simulink model "Filter_attivo"  (R2016b)
settings: Solver=ode23t  StartTime=0.0  StopTime=2.4  MaxStep=1e-4  RelTol=1e-3  EnableMultiTasking=on
values from neighbouring files (symbols this model uses):
  ampiezza_rete = 150/sqrt(3)    [Data.m]    (also in taratura.m)
  C = 2.2e-3    (= 0.0022)    [Data.m]
  C_raddr = 600e-6    (= 0.0006)    [Data.m]
  f = 50    [Data.m]    (also in Spettro_complesso.m = bar(-fp((26:25:25000-25)),PyTHD(length(PyTHD)-1:-1:length(Py)
  f_am = 500    [Data.m]
  h = Lagrange_coef(f,1/Tc)    [Data.m]    (also in Lagrange_coef.m = NaN(4,round(fc/f1*0.5)))
  h_rit = Lagrange_coef_rit(1.5)    [Data.m]
  k_interno = 0.99    [tuning.m]
  k_par_AM = 10    [Data.m]
  ki_PI = 0.2    [Data.m]
  ki_PLL = 1000    [Data.m]
  ki_ris = 47.5*2    (= 95)    [Data.m]
  kp_PI = 1.57    [Data.m]
  kp_PLL = 0.9    [Data.m]
  kp_ris = 47.5*0.089*2    (= 8.455)    [Data.m]
  L_disaccoppiamento = 2*1.18e-3    (= 0.00236)    [Data.m]    (also in taratura.m)
  L_rete = 4e-3    (= 0.004)    [Data.m]    (also in tuning.m)
  max_PI = 8    [Data.m]
  max_PLL = 1000    [Data.m]
  min_PI = -8    [Data.m]
  min_PLL = -1000    [Data.m]
  Notch_z = 1-Peaking_z    [Data.m]
  Notch_z_AM1 = 1-Peaking_z_AM1    [Notch.m]
  peak_rete = Peaking(f,1/Tc,0.1)    [Data.m]
  Peaking_dir1_d = c2d(Peaking_dir1_s,1/fs,'tustin')    [semipeaking.m]
  pendenza = 1000    [Data.m]
  R_carico = 50    [Data.m]
  R_disaccoppiamento = 2*13e-3    (= 0.026)    [Data.m]    (also in taratura.m)
  R_raddr = 60    [Data.m]
  R_rete = 100e-3    (= 0.1)    [Data.m]    (also in tuning.m = 0.01)
  T = 20e-3    (= 0.02)    [Data.m]    (also in tuning.m)
  tau_filtro_Vdc_ref = 0.15    [Data.m]
  Tc = 1/10000    (= 0.0001)    [Data.m]    (also in taratura.m; tuning.m)
  Vdc_ref = 200    [Data.m]    (also in taratura.m)
  w_filtro = 2*pi*f_taglio    (= 56548.6677646)    [Data.m]
undefined symbols (not defined in the file or in its folder): DiscIntNeverNeededParam, k_par, k_ser, Notch_z_AM1_5, Notch_z_AM1_7, Notch_z_AM2_5, Notch_z_AM2_7, Peaking_inv_d, plecs, Q_inv
libraries: powerlib x54, simulink x8, powerlib_extras x4, powerlib_meascontrol x2
(part 3 of 5)

== system Filter_attivo/Controllo tensione/Controllo ripetitivo/Notch Prima Armonica/D ==
  ab(c) : Inport
  Gain : Gain  Gain=[1 0; 1/sqrt(3) 2/sqrt(3)]  Multiplication=Matrix(K*u)
  dq(0) : Outport
  wires:
  Gain/1 -> dq(0)/1
  ab(c)/1 -> Gain/1

== system Filter_attivo/Controllo tensione/Controllo ripetitivo/Notch Prima Armonica/Filtro notch prima armonica  ==
  ir : Inport
  Discrete Transfer Fcn : DiscreteTransferFcn  Numerator=Notch_z.num{1,1}  Denominator=Notch_z.den{1,1}
  irh : Outport
  wires:
  ir/1 -> Discrete Transfer Fcn/1
  Discrete Transfer Fcn/1 -> irh/1

== system Filter_attivo/Controllo tensione/Controllo ripetitivo/Notch Prima Armonica/Filtro notch prima armonica 1 ==
  ir : Inport
  Discrete Transfer Fcn : DiscreteTransferFcn  Numerator=Notch_z.num{1,1}  Denominator=Notch_z.den{1,1}
  irh : Outport
  wires:
  Discrete Transfer Fcn/1 -> irh/1
  ir/1 -> Discrete Transfer Fcn/1

== system Filter_attivo/Rete/generatore diretta e inversa/Scope1/ InputMux  ==
  In1 : Inport
  Convert1 : DataTypeConversion  SaturateOnIntegerOverflow=on  RndMeth=Zero
  Mux : Mux  Inputs=1
  Out : Outport
  wires:
  Mux/1 -> Out/1
  In1/1 -> Convert1/1
  Convert1/1 -> Mux/1

== system Filter_attivo/Controllo tensione/Controllo PR 10 kHz/Controllo risonante/Contributo controllo risonante fondamentale/PIR_tustin_prewarp ==
  errore_d : Inport
  errore_q : Inport  Port=2
  Vdc : Inport  Port=3
  Enable : EnablePort  StatesWhenEnabling=reset
  Constant : Constant  Value=kp_ris
  Constant1 : Constant  Value=kr_ris
  Constant2 : Constant  Value=Tc
  Constant3 : Constant  Value=delta
  Constant4 : Constant  Value=w_ris
  Gain : Gain  Gain=-1
  MATLAB Function : MATLAB Function  TreatAsAtomicUnit=on
  MATLAB Function1 : MATLAB Function  TreatAsAtomicUnit=on
  vf1_d : Outport
  vfq_q : Outport  Port=2
  wires:
  errore_d/1 -> MATLAB Function/1(error)
  Constant/1 -> MATLAB Function1/2(kp), MATLAB Function/2(kp)
  Constant1/1 -> MATLAB Function1/3(ki), MATLAB Function/3(ki)
  Vdc/1 -> Gain/1, MATLAB Function1/5(max), MATLAB Function/5(max)
  Gain/1 -> MATLAB Function1/4(min), MATLAB Function/4(min)
  Constant2/1 -> MATLAB Function1/6(Tc), MATLAB Function/6(Tc)
  Constant3/1 -> MATLAB Function1/7(delta), MATLAB Function/7(delta)
  Constant4/1 -> MATLAB Function/8(w0)
  MATLAB Function/1(out) -> vf1_d/1
  MATLAB Function1/1(out) -> vfq_q/1
  errore_q/1 -> MATLAB Function1/8(w0), MATLAB Function1/1(error)

== system Filter_attivo/Controllo tensione/Controllo PR 10 kHz/Controllo risonante/Contributo controllo risonante fondamentale/PI_risonante ==
  note: Questa è la discretizzazione di un PIR alla frequenza w0 della fondamentale (314 rad/s)
      | utlizzando la discretizzazione di Tustin con Prewarp
  In1 : Inport
  In2 : Inport  Port=2
  Enable : EnablePort  StatesWhenEnabling=reset
  Add : Sum
  Demux : Demux  Outputs=2
  Demux1 : Demux  Outputs=2
  Discrete Transfer Fcn2 : DiscreteTransferFcn  Numerator=[sin(Tc*2*pi*f) 0 -sin(Tc*2*pi*f)]  Denominator=[2*2*pi*f -2*2*2*pi*f*cos(Tc*2*pi*f) 2*2*pi*f]
  Discrete Transfer Fcn3 : DiscreteTransferFcn  Numerator=[sin(Tc*2*pi*f) 0 -sin(Tc*2*pi*f)]  Denominator=[2*2*pi*f -2*2*2*pi*f*cos(Tc*2*pi*f) 2*2*pi*f]
  Gain : Gain  Gain=ki_ris
  Gain1 : Gain  Gain=kp_ris
  Mux : Mux  Inputs=2
  Mux1 : Mux  Inputs=2
  Out1 : Outport
  Out2 : Outport  Port=2
  wires:
  Mux/1 -> Gain1/1, Gain/1
  In1/1 -> Mux/1
  In2/1 -> Mux/2
  Demux/1 -> Out1/1
  Demux/2 -> Out2/1
  Add/1 -> Demux/1
  Mux1/1 -> Add/2
  Gain/1 -> Demux1/1
  Gain1/1 -> Add/1
  Demux1/1 -> Discrete Transfer Fcn2/1
  Demux1/2 -> Discrete Transfer Fcn3/1
  Discrete Transfer Fcn2/1 -> Mux1/1
  Discrete Transfer Fcn3/1 -> Mux1/2

== system Filter_attivo/Controllo tensione/Controllo PR 10 kHz/Controllo risonante/FILTRO peaking inversa_prima/Scope ==
  1 : Inport
  " InputMux " : Subsystem
      mask Display: disp('Mux')
  " S-Function " : S-Function  FunctionName=plecs  SFunctionDeploymentMode=off  EnableBusSupport=off
  wires:
  1/1 -> " InputMux "/1(In1)
  " InputMux "/1(Out) -> " S-Function "/1

== system Filter_attivo/Controllo tensione/Controllo PR 10 kHz/PLL_tempo_discreto/Subsystem/FILTRO peaking diretta_prima ==
  In2 : Inport
  Demux : Demux  Outputs=2
  Discrete Transfer Fcn : DiscreteTransferFcn  Numerator=cell2mat(Peaking_dir1_d(1,1).Num)  Denominator=cell2mat(Peaking_dir1_d(1,1).Den)
  Discrete Transfer Fcn1 : DiscreteTransferFcn  Numerator=cell2mat(Peaking_dir1_d(1,2).Num)  Denominator=cell2mat(Peaking_dir1_d(1,2).Den)
  Discrete Transfer Fcn2 : DiscreteTransferFcn  Numerator=cell2mat(Peaking_dir1_d(2,1).Num)  Denominator=cell2mat(Peaking_dir1_d(2,1).Den)
  Discrete Transfer Fcn3 : DiscreteTransferFcn  Numerator=cell2mat(Peaking_dir1_d(2,2).Num)  Denominator=cell2mat(Peaking_dir1_d(2,2).Den)
  Mux1 : Mux  Inputs=2
  Scope : Subsystem  LoadFcn=plecs('sl', 300);  InitFcn=plecs('sl', 314);  StartFcn=plecs('sl', 308);  StopFcn=plecs('sl', 309);  mask{Settings=<binary blob, 216 chars, not shown>}
      mask init:
      | plecs('sl', 315);
      settings: CopyFcn=plecs('sl', 303);  DeleteFcn=plecs('sl', 305);  UndoDeleteFcn=plecs('sl', 306);  PreSaveFcn=plecs('sl', 311);  NameChangeFcn=plecs('sl', 310);  DestroyFcn=plecs('sl', 307);  OpenFcn=plecs('sl', 302);  ErrorFcn=plerrorfcn
      mask Display: plot([0.1 0.9 0.9 0.1 0.1], [0.9 0.9 0.5 0.5 0.9])
  Sum3 : Sum  Inputs=|++
  Sum4 : Sum  Inputs=|++
  Out1 : Outport
  wires:
  Demux/1 -> Discrete Transfer Fcn2/1, Discrete Transfer Fcn/1
  Demux/2 -> Discrete Transfer Fcn1/1, Discrete Transfer Fcn3/1
  Discrete Transfer Fcn2/1 -> Sum4/1
  Sum4/1 -> Mux1/2
  Mux1/1 -> Out1/1
  Sum3/1 -> Mux1/1, Scope/1(1)
  Discrete Transfer Fcn/1 -> Sum3/1
  Discrete Transfer Fcn1/1 -> Sum3/2
  In2/1 -> Demux/1
  Discrete Transfer Fcn3/1 -> Sum4/2

== system Filter_attivo/Controllo tensione/Controllo PR 10 kHz/PLL_tempo_discreto/Subsystem/notch_prima_tensione ==
  In1 : Inport
  FILTRO peaking diretta_prima : Subsystem
  Sum : Sum  Inputs=|+-
  Out1 : Outport
  wires:
  In1/1 -> FILTRO peaking diretta_prima/1(In2), Sum/1
  Sum/1 -> Out1/1
  FILTRO peaking diretta_prima/1(Out1) -> Sum/2

== system Filter_attivo/Controllo tensione/Controllo PR 10 kHz/controllo /Scope/ InputMux  ==
  In1 : Inport
  Convert1 : DataTypeConversion  SaturateOnIntegerOverflow=on  RndMeth=Zero
  Mux : Mux  Inputs=1
  Out : Outport
  wires:
  Convert1/1 -> Mux/1
  In1/1 -> Convert1/1
  Mux/1 -> Out/1

== system Filter_attivo/Controllo tensione/Controllo PR 10 kHz/controllo /Scope1/ InputMux  ==
  In1 : Inport
  Convert1 : DataTypeConversion  SaturateOnIntegerOverflow=on  RndMeth=Zero
  Mux : Mux  Inputs=1
  Out : Outport
  wires:
  Mux/1 -> Out/1
  In1/1 -> Convert1/1
  Convert1/1 -> Mux/1

== system Filter_attivo/Controllo tensione/Controllo PR 10 kHz/controllo /Scope2/ InputMux  ==
  In1 : Inport
  Convert1 : DataTypeConversion  SaturateOnIntegerOverflow=on  RndMeth=Zero
  Mux : Mux  Inputs=1
  Out : Outport
  wires:
  Convert1/1 -> Mux/1
  In1/1 -> Convert1/1
  Mux/1 -> Out/1

== system Filter_attivo/Controllo tensione/Controllo PR 10 kHz/controllo /Scope3/ InputMux  ==
  In1 : Inport
  Convert1 : DataTypeConversion  SaturateOnIntegerOverflow=on  RndMeth=Zero
  Mux : Mux  Inputs=1
  Out : Outport
  wires:
  Mux/1 -> Out/1
  In1/1 -> Convert1/1
  Convert1/1 -> Mux/1

== system Filter_attivo/Controllo tensione/Controllo ripetitivo/Controllo ripetitivo/Regolatore ripetitivo/ Ripetitivo sincrono ==
  note: A
  ir : Inport
  Add : Sum
  Delay1 : Delay  DelayLength=rit
  Delay2 : Delay  DelayLength=round((1/ro/f/Tc)-rit-1)
  Gain1 : Gain
  Gain2 : Gain  Gain=k_ser_
  Scope : Subsystem  LoadFcn=plecs('sl', 300);  InitFcn=plecs('sl', 314);  StartFcn=plecs('sl', 308);  StopFcn=plecs('sl', 309);  mask{Settings=<binary blob, 384 chars, not shown>}
      mask init:
      | plecs('sl', 315);
      settings: CopyFcn=plecs('sl', 303);  DeleteFcn=plecs('sl', 305);  UndoDeleteFcn=plecs('sl', 306);  PreSaveFcn=plecs('sl', 311);  NameChangeFcn=plecs('sl', 310);  DestroyFcn=plecs('sl', 307);  OpenFcn=plecs('sl', 302);  ErrorFcn=plerrorfcn
      mask Display: plot([0.1 0.9 0.9 0.1 0.1], [0.9 0.9 0.5 0.5 0.9])
  Sum : Sum  Inputs=|--
  ritardo di 1.5 : DiscreteFir  Coefficients=[0.5 0. 0.5]
  Out : Outport
  wires:
  Gain2/1 -> Scope/2(2), Add/2
  Add/1 -> Scope/3(3), Out/1
  Delay1/1 -> Gain1/1
  Delay2/1 -> ritardo di 1.5/1
  Sum/1 -> Delay2/1
  Gain1/1 -> Sum/2
  ritardo di 1.5/1 -> Gain2/1, Delay1/1
  ir/1 -> Add/1, Sum/1

== system Filter_attivo/Controllo tensione/Controllo ripetitivo/Controllo ripetitivo/Regolatore ripetitivo/ Ripetitivo sincrono feedforward ==
  note: B
  note: A
  ir : Inport
  Delay2 : Delay  DelayLength=round((1/ro/f/Tc)-1)
  Delay3 : Delay  DelayLength=round((1/f/Tc/ro)-rit)
  Gain2 : Gain  Gain=k_ser_
  Q : DiscreteFir  Coefficients=[0.25 0.5 0.25]
  Sum : Sum  Inputs=|--
  Sum1 : Sum  Inputs=+-|
  Sum2 : Sum
  Out : Outport
  wires:
  Sum2/1 -> Out/1
  Gain2/1 -> Sum2/2
  Delay3/1 -> Gain2/1
  Sum1/1 -> Delay3/1
  ir/1 -> Sum/1, Sum2/1
  Q/1 -> Sum1/2, Sum/2
  Delay2/1 -> Q/1
  Sum/1 -> Delay2/1, Sum1/1

== system Filter_attivo/Controllo tensione/Controllo ripetitivo/Controllo ripetitivo/Regolatore ripetitivo/ buffer intero fase zero ==
  note: A
  e : Inport
  Add : Sum
  Delay1 : Delay  DelayLength=rit
  Delay2 : Delay  DelayLength=round((1/ro/f/Tc)-1-rit)
  Gain1 : Gain
  Gain2 : Gain  Gain=k_serie
  Q : DiscreteFir  Coefficients=[0.05 0.9 0.05]
  Scope : Subsystem  LoadFcn=plecs('sl', 300);  InitFcn=plecs('sl', 314);  StartFcn=plecs('sl', 308);  StopFcn=plecs('sl', 309);  mask{Settings=<binary blob, 424 chars, not shown>}
      mask init:
      | plecs('sl', 315);
      settings: CopyFcn=plecs('sl', 303);  DeleteFcn=plecs('sl', 305);  UndoDeleteFcn=plecs('sl', 306);  PreSaveFcn=plecs('sl', 311);  NameChangeFcn=plecs('sl', 310);  DestroyFcn=plecs('sl', 307);  OpenFcn=plecs('sl', 302);  ErrorFcn=plerrorfcn
      mask Display: plot([0.1 0.9 0.9 0.1 0.1], [0.9 0.9 0.5 0.5 0.9])
  Subsystem : Subsystem  mask{f_disturbo=265, g_disturbo=0.1}
      mask prompts: f_disturbo "frequeza [Hz] del disturbo"; g_disturbo "valore [pu] del disturbo"
  Sum : Sum  Inputs=|++
  Out : Outport
  wires:
  Gain1/1 -> Sum/2
  Sum/1 -> Delay2/1
  Delay2/1 -> Q/1
  Delay1/1 -> Gain1/1
  e/1 -> Subsystem/1(errore)
  Add/1 -> Out/1, Scope/3(3)
  Gain2/1 -> Scope/2(2), Add/2
  Subsystem/1(errore+disturbo) -> Scope/1(1), Sum/1, Add/1
  Q/1 -> Delay1/1, Gain2/1

== system Filter_attivo/Controllo tensione/Controllo ripetitivo/Controllo ripetitivo/Regolatore ripetitivo/ buffer intero fase zero1 ==
  note: A
  e : Inport
  Add : Sum
  Delay2 : Delay  DelayLength=round((1/ro/f/Tc)-4)
  Gain1 : Gain
  Gain2 : Gain  Gain=k_serie
  Q : DiscreteFir  Coefficients=[0.05 0.9 0.05]
  Q1 : DiscreteFir  Coefficients=[-0.0625 0.5625 0.5625 -0.0625]
  Q2 : DiscreteFir  Coefficients=[-0.0625 0.5625 0.5625 -0.0625]
  Scope : Subsystem  LoadFcn=plecs('sl', 300);  InitFcn=plecs('sl', 314);  StartFcn=plecs('sl', 308);  StopFcn=plecs('sl', 309);  mask{Settings=<binary blob, 424 chars, not shown>}
      mask init:
      | plecs('sl', 315);
      settings: CopyFcn=plecs('sl', 303);  DeleteFcn=plecs('sl', 305);  UndoDeleteFcn=plecs('sl', 306);  PreSaveFcn=plecs('sl', 311);  NameChangeFcn=plecs('sl', 310);  DestroyFcn=plecs('sl', 307);  OpenFcn=plecs('sl', 302);  ErrorFcn=plerrorfcn
      mask Display: plot([0.1 0.9 0.9 0.1 0.1], [0.9 0.9 0.5 0.5 0.9])
  Sum : Sum  Inputs=|++
  Out : Outport
  wires:
  Q/1 -> Q2/1
  e/1 -> Sum/1, Scope/1(1), Add/1
  Gain2/1 -> Add/2, Scope/2(2)
  Add/1 -> Scope/3(3), Out/1
  Q1/1 -> Gain1/1
  Delay2/1 -> Q/1
  Sum/1 -> Delay2/1
  Gain1/1 -> Sum/2
  Q2/1 -> Q1/1, Gain2/1

== system Filter_attivo/Controllo tensione/Controllo ripetitivo/Controllo ripetitivo/Regolatore ripetitivo/ buffer intero feedforward ==
  note: A
  note: B
  e : Inport
  Delay 1 : Delay  DelayLength=round((1/ro/f/Tc)-1)
  Delay 2 : Delay  DelayLength=round((1/ro/f/Tc)-rit)
  Gain2 : Gain  Gain=k_serie
  Q : DiscreteFir  Coefficients=[0.05 0.9 0.05]
  Scope : Subsystem  LoadFcn=plecs('sl', 300);  InitFcn=plecs('sl', 314);  StartFcn=plecs('sl', 308);  StopFcn=plecs('sl', 309);  mask{Settings=<binary blob, 892 chars, not shown>}
      mask init:
      | plecs('sl', 315);
      settings: CopyFcn=plecs('sl', 303);  DeleteFcn=plecs('sl', 305);  UndoDeleteFcn=plecs('sl', 306);  PreSaveFcn=plecs('sl', 311);  NameChangeFcn=plecs('sl', 310);  DestroyFcn=plecs('sl', 307);  OpenFcn=plecs('sl', 302);  ErrorFcn=plerrorfcn
      mask Display: plot([0.1 0.9 0.9 0.1 0.1], [0.9 0.9 0.5 0.5 0.9])
  Scope1 : Subsystem  LoadFcn=plecs('sl', 300);  InitFcn=plecs('sl', 314);  StartFcn=plecs('sl', 308);  StopFcn=plecs('sl', 309);  mask{Settings=<binary blob, 892 chars, not shown>}
      mask init:
      | plecs('sl', 315);
      settings: CopyFcn=plecs('sl', 303);  DeleteFcn=plecs('sl', 305);  UndoDeleteFcn=plecs('sl', 306);  PreSaveFcn=plecs('sl', 311);  NameChangeFcn=plecs('sl', 310);  DestroyFcn=plecs('sl', 307);  OpenFcn=plecs('sl', 302);  ErrorFcn=plerrorfcn
      mask Display: plot([0.1 0.9 0.9 0.1 0.1], [0.9 0.9 0.5 0.5 0.9])
  Subsystem : Subsystem  mask{f_disturbo=275, g_disturbo=0.3}
      mask prompts: f_disturbo "frequeza [Hz] del disturbo"; g_disturbo "valore [pu] del disturbo"
  Sum : Sum  Inputs=|++
  Sum1 : Sum  Inputs=++|
  Sum2 : Sum
  Out : Outport
  wires:
  Sum/1 -> Sum1/1, Delay 1/1
  Delay 1/1 -> Q/1
  Q/1 -> Sum/2, Sum1/2
  e/1 -> Scope1/1(1), Subsystem/1(errore)
  Sum1/1 -> Delay 2/1
  Delay 2/1 -> Gain2/1
  Gain2/1 -> Sum2/2
  Sum2/1 -> Out/1
  Subsystem/1(errore+disturbo) -> Sum2/1, Sum/1, Scope/1(1)

== system Filter_attivo/Controllo tensione/Controllo ripetitivo/Controllo ripetitivo/Regolatore ripetitivo/ buffer metà fase zero ==
  note: A
  e : Inport
  Add : Sum
  Delay1 : Delay  DelayLength=rit
  Delay2 : Delay  DelayLength=round((1/ro/f/Tc)-1-rit)
  Gain1 : Gain
  Gain2 : Gain  Gain=k_serie
  Q : DiscreteFir  Coefficients=[0.05 0.9 0.05]
  Scope : Subsystem  LoadFcn=plecs('sl', 300);  InitFcn=plecs('sl', 314);  StartFcn=plecs('sl', 308);  StopFcn=plecs('sl', 309);  mask{Settings=<binary blob, 424 chars, not shown>}
      mask init:
      | plecs('sl', 315);
      settings: CopyFcn=plecs('sl', 303);  DeleteFcn=plecs('sl', 305);  UndoDeleteFcn=plecs('sl', 306);  PreSaveFcn=plecs('sl', 311);  NameChangeFcn=plecs('sl', 310);  DestroyFcn=plecs('sl', 307);  OpenFcn=plecs('sl', 302);  ErrorFcn=plerrorfcn
      mask Display: plot([0.1 0.9 0.9 0.1 0.1], [0.9 0.9 0.5 0.5 0.9])
  Sum : Sum  Inputs=|--
  Out : Outport
  wires:
  Gain1/1 -> Sum/2
  Sum/1 -> Delay2/1
  Delay2/1 -> Q/1
  Delay1/1 -> Gain1/1
  e/1 -> Scope/1(1), Sum/1, Add/1
  Add/1 -> Out/1, Scope/3(3)
  Q/1 -> Gain2/1, Delay1/1
  Gain2/1 -> Scope/2(2), Add/2

== system Filter_attivo/Controllo tensione/Controllo ripetitivo/Controllo ripetitivo/Regolatore ripetitivo/ buffer metà feedforward ==
  note: A
  note: B
  e : Inport
  Delay2 : Delay  DelayLength=round((1/ro/f/Tc)-1)
  Delay3 : Delay  DelayLength=round((1/f/Tc/ro)-rit)
  Gain2 : Gain  Gain=k_serie
  Q : DiscreteFir  Coefficients=[0.05 0.9 0.05]
  Scope : Subsystem  LoadFcn=plecs('sl', 300);  InitFcn=plecs('sl', 314);  StartFcn=plecs('sl', 308);  StopFcn=plecs('sl', 309);  mask{Settings=<binary blob, 876 chars, not shown>}
      mask init:
      | plecs('sl', 315);
      settings: CopyFcn=plecs('sl', 303);  DeleteFcn=plecs('sl', 305);  UndoDeleteFcn=plecs('sl', 306);  PreSaveFcn=plecs('sl', 311);  NameChangeFcn=plecs('sl', 310);  DestroyFcn=plecs('sl', 307);  OpenFcn=plecs('sl', 302);  ErrorFcn=plerrorfcn
      mask Display: plot([0.1 0.9 0.9 0.1 0.1], [0.9 0.9 0.5 0.5 0.9])
  Subsystem : Subsystem  mask{f_disturbo=275, g_disturbo=0.1}
      mask prompts: f_disturbo "frequeza [Hz] del disturbo"; g_disturbo "valore [pu] del disturbo"
  Sum : Sum  Inputs=|--
  Sum1 : Sum  Inputs=+-|
  Sum2 : Sum
  Out : Outport
  wires:
  Sum2/1 -> Out/1
  Gain2/1 -> Sum2/2
  Delay3/1 -> Gain2/1
  Sum1/1 -> Delay3/1
  Q/1 -> Sum/2, Sum1/2
  Delay2/1 -> Q/1
  Sum/1 -> Delay2/1, Sum1/1
  Subsystem/1(errore+disturbo) -> Sum2/1, Sum/1, Scope/1(1)
  e/1 -> Subsystem/1(errore)

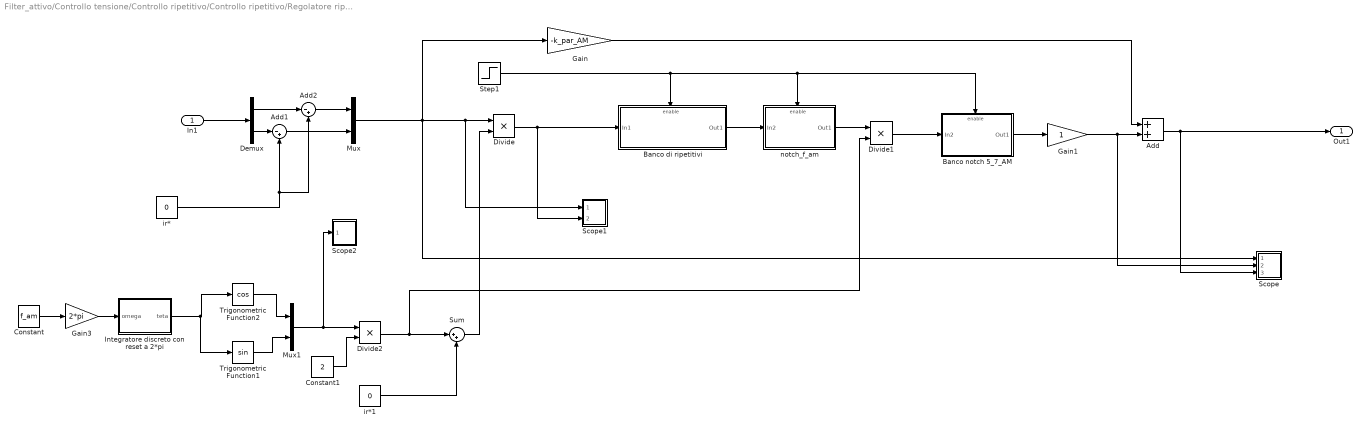
== system Filter_attivo/Controllo tensione/Controllo ripetitivo/Controllo ripetitivo/Regolatore ripetitivo/Ripetitivo Modulazione AM ==
  In1 : Inport
  Add : Sum
  Add1 : Sum  Inputs=|-+
  Add2 : Sum  Inputs=|-+
  Banco di ripetitivi : Subsystem
  Banco notch 5_7_AM : Subsystem
  Constant : Constant  Value=f_am
  Constant1 : Constant  Value=2
  Demux : Demux  Outputs=2
  Divide : Product  Inputs=**
  Divide1 : Product  Inputs=**
  Divide2 : Product  Inputs=**
  Gain : Gain  Gain=-k_par_AM
  Gain1 : Gain
  Gain3 : Gain  Gain=2*pi
  Integratore discreto con reset a 2*pi : Subsystem
  Mux : Mux  Inputs=2
  Mux1 : Mux  Inputs=2
  Scope : Subsystem  LoadFcn=plecs('sl', 300);  InitFcn=plecs('sl', 314);  StartFcn=plecs('sl', 308);  StopFcn=plecs('sl', 309);  mask{Settings=<binary blob, 424 chars, not shown>}
      mask init:
      | plecs('sl', 315);
      settings: CopyFcn=plecs('sl', 303);  DeleteFcn=plecs('sl', 305);  UndoDeleteFcn=plecs('sl', 306);  PreSaveFcn=plecs('sl', 311);  NameChangeFcn=plecs('sl', 310);  DestroyFcn=plecs('sl', 307);  OpenFcn=plecs('sl', 302);  ErrorFcn=plerrorfcn
      mask Display: plot([0.1 0.9 0.9 0.1 0.1], [0.9 0.9 0.5 0.5 0.9])
  Scope1 : Subsystem  LoadFcn=plecs('sl', 300);  InitFcn=plecs('sl', 314);  StartFcn=plecs('sl', 308);  StopFcn=plecs('sl', 309);  mask{Settings=<binary blob, 300 chars, not shown>}
      mask init:
      | plecs('sl', 315);
      settings: CopyFcn=plecs('sl', 303);  DeleteFcn=plecs('sl', 305);  UndoDeleteFcn=plecs('sl', 306);  PreSaveFcn=plecs('sl', 311);  NameChangeFcn=plecs('sl', 310);  DestroyFcn=plecs('sl', 307);  OpenFcn=plecs('sl', 302);  ErrorFcn=plerrorfcn
      mask Display: plot([0.1 0.9 0.9 0.1 0.1], [0.9 0.9 0.5 0.5 0.9])
  Scope2 : Subsystem  LoadFcn=plecs('sl', 300);  InitFcn=plecs('sl', 314);  StartFcn=plecs('sl', 308);  StopFcn=plecs('sl', 309);  mask{Settings=<binary blob, 216 chars, not shown>}
      mask init:
      | plecs('sl', 315);
      settings: CopyFcn=plecs('sl', 303);  DeleteFcn=plecs('sl', 305);  UndoDeleteFcn=plecs('sl', 306);  PreSaveFcn=plecs('sl', 311);  NameChangeFcn=plecs('sl', 310);  DestroyFcn=plecs('sl', 307);  OpenFcn=plecs('sl', 302);  ErrorFcn=plerrorfcn
      mask Display: plot([0.1 0.9 0.9 0.1 0.1], [0.9 0.9 0.5 0.5 0.9])
  Step1 : Step  Time=0.45
  Sum : Sum  Inputs=|++
  Trigonometric Function1 : Trigonometry
  Trigonometric Function2 : Trigonometry  Operator=cos
  ir* : Constant  Value=0
  ir*1 : Constant  Value=0
  notch_f_am : Subsystem
  Out1 : Outport
  wires:
  Gain/1 -> Add/1
  Constant/1 -> Gain3/1
  Gain3/1 -> Integratore discreto con reset a 2*pi/1(omega)
  Add1/1 -> Mux/2
  ir*/1 -> Add1/2, Add2/2
  Add/1 -> Out1/1, Scope/3(3)
  Demux/1 -> Add2/1
  In1/1 -> Demux/1
  Add2/1 -> Mux/1
  Demux/2 -> Add1/1
  Mux/1 -> Scope/1(1), Gain/1, Scope1/1(1), Divide/1
  Divide1/1 -> Banco notch 5_7_AM/1(In2)
  Banco notch 5_7_AM/1(Out1) -> Gain1/1
  Integratore discreto con reset a 2*pi/1(teta) -> Trigonometric Function1/1, Trigonometric Function2/1
  Trigonometric Function2/1 -> Mux1/1
  Trigonometric Function1/1 -> Mux1/2
  Mux1/1 -> Scope2/1(1), Divide2/1
  Constant1/1 -> Divide2/2
  Step1/1 -> notch_f_am/Enable, Banco notch 5_7_AM/Enable, Banco di ripetitivi/Enable
  Gain1/1 -> Scope/2(2), Add/2
  Divide/1 -> Banco di ripetitivi/1(In1), Scope1/2(2)
  Divide2/1 -> Divide1/2, Sum/1
  ir*1/1 -> Sum/2
  Sum/1 -> Divide/2
  Banco di ripetitivi/1(Out1) -> notch_f_am/1(In2)
  notch_f_am/1(Out1) -> Divide1/1

== system Filter_attivo/Controllo tensione/Controllo ripetitivo/Controllo ripetitivo/Regolatore ripetitivo/Scope ==
  1 : Inport
  " InputMux " : Subsystem
      mask Display: disp('Mux')
  " S-Function " : S-Function  FunctionName=plecs  SFunctionDeploymentMode=off  EnableBusSupport=off
  wires:
  1/1 -> " InputMux "/1(In1)
  " InputMux "/1(Out) -> " S-Function "/1

== system Filter_attivo/Controllo tensione/Controllo ripetitivo/Controllo ripetitivo/Regolatore ripetitivo/T ==
  dq : Inport
  teta : Inport  Port=2
  Demux : Demux  Outputs=2
  Fcn : Fcn  Expr=cos(u[3])*u[1]+sin(u[3])*u[2]
  Fcn1 : Fcn  Expr=-sin(u[3])*u[1]+cos(u[3])*u[2]
  Gain8 : Gain
  Mux : Mux  Inputs=3
  Mux1 : Mux  Inputs=2
  dq(teta) : Outport
  wires:
  dq/1 -> Demux/1
  Demux/1 -> Mux/1
  Demux/2 -> Mux/2
  Mux/1 -> Fcn/1, Fcn1/1
  Fcn/1 -> Mux1/1
  Fcn1/1 -> Mux1/2
  Mux1/1 -> dq(teta)/1
  teta/1 -> Gain8/1
  Gain8/1 -> Mux/3

== system Filter_attivo/Controllo tensione/Controllo ripetitivo/Controllo ripetitivo/Regolatore ripetitivo/T1 ==
  dq : Inport
  teta : Inport  Port=2
  Demux : Demux  Outputs=2
  Fcn : Fcn  Expr=cos(u[3])*u[1]+sin(u[3])*u[2]
  Fcn1 : Fcn  Expr=-sin(u[3])*u[1]+cos(u[3])*u[2]
  Gain8 : Gain
  Mux : Mux  Inputs=3
  Mux1 : Mux  Inputs=2
  dq(teta) : Outport
  wires:
  dq/1 -> Demux/1
  Demux/1 -> Mux/1
  Demux/2 -> Mux/2
  Mux/1 -> Fcn/1, Fcn1/1
  Fcn/1 -> Mux1/1
  Fcn1/1 -> Mux1/2
  Mux1/1 -> dq(teta)/1
  teta/1 -> Gain8/1
  Gain8/1 -> Mux/3

== system Filter_attivo/Controllo tensione/Controllo ripetitivo/Controllo ripetitivo/Regolatore ripetitivo/T_inversa ==
  dq(teta) : Inport
  teta : Inport  Port=2
  Demux : Demux  Outputs=2
  Fcn : Fcn  Expr=cos(u[3])*u[1]+sin(u[3])*u[2]
  Fcn1 : Fcn  Expr=-sin(u[3])*u[1]+cos(u[3])*u[2]
  Gain8 : Gain  Gain=-1
  Mux : Mux  Inputs=3
  Mux1 : Mux  Inputs=2
  dq(0) : Outport
  wires:
  dq(teta)/1 -> Demux/1
  Demux/1 -> Mux/1
  Demux/2 -> Mux/2
  Mux/1 -> Fcn/1, Fcn1/1
  Fcn/1 -> Mux1/1
  Fcn1/1 -> Mux1/2
  Mux1/1 -> dq(0)/1
  teta/1 -> Gain8/1
  Gain8/1 -> Mux/3

== system Filter_attivo/Controllo tensione/Controllo ripetitivo/Controllo ripetitivo/Regolatore ripetitivo/T_inversa1 ==
  dq(teta) : Inport
  teta : Inport  Port=2
  Demux : Demux  Outputs=2
  Fcn : Fcn  Expr=cos(u[3])*u[1]+sin(u[3])*u[2]
  Fcn1 : Fcn  Expr=-sin(u[3])*u[1]+cos(u[3])*u[2]
  Gain8 : Gain  Gain=-1
  Mux : Mux  Inputs=3
  Mux1 : Mux  Inputs=2
  dq(0) : Outport
  wires:
  dq(teta)/1 -> Demux/1
  Demux/1 -> Mux/1
  Demux/2 -> Mux/2
  Mux/1 -> Fcn/1, Fcn1/1
  Fcn/1 -> Mux1/1
  Fcn1/1 -> Mux1/2
  Mux1/1 -> dq(0)/1
  teta/1 -> Gain8/1
  Gain8/1 -> Mux/3

== system Filter_attivo/Controllo tensione/Controllo ripetitivo/Controllo ripetitivo/Regolatore ripetitivo/vecchi controlli ==
  In1 : Inport
  In2 : Inport  Port=2
  In3 : Inport  Port=3
  In4 : Inport  Port=4
  In5 : Inport  Port=5
  " Ripetitivo buffer intero" : Subsystem  mask{ro=1, rit=4, k_serie=10.1, k_parallelo=10}
      mask prompts: ro "Riduzione Buffer"; rit "Cicli compensati inverter"
  " Ripetitivo buffer intero1.5 di ritardo" : Subsystem  mask{ro=1, rit=0, k_serie=6, k_parallelo=2.5}
      mask prompts: ro "Riduzione Buffer"; rit "Ulteriori cicli compensati"
  " Ripetitivo stazionario" : Subsystem  Commented=on  mask{ro=2, rit=3}
      mask prompts: ro "Riduzione Buffer"; rit "Cicli compensati inverter"
  " buffer intero mattavelli buchi amplificati" : Subsystem  mask{ro=1, rit=2, k_serie=5}
      mask prompts: ro "Riduzione Buffer"; rit "cicli compensati"
  "Generatore step " : Subsystem  mask{k_serie_partenza=5, passo_t=0.1, passo_y=0.5}
      mask prompts: k_serie_partenza "partenza della costante"; passo_t "step dei tempi"; passo_y "step di costante"
  Ripetitivo Modulazione AM1 : Subsystem  Commented=on
  Out1 : Outport
  Out2 : Outport  Port=2
  Out3 : Outport  Port=3
  Out4 : Outport  Port=4
  Out5 : Outport  Port=5
  wires:
  " Ripetitivo buffer intero"/1(Out) -> Out3/1
  In4/1 -> Ripetitivo Modulazione AM1/1(In1)
  In3/1 -> " Ripetitivo buffer intero"/1(ir)
  In5/1 -> " Ripetitivo stazionario"/1(ir)
  " Ripetitivo stazionario"/1(Out) -> Out5/1
  Ripetitivo Modulazione AM1/1(Out1) -> Out4/1
  In2/1 -> " Ripetitivo buffer intero1.5 di ritardo"/1(ir)
  " Ripetitivo buffer intero1.5 di ritardo"/1(Out) -> Out2/1
  " buffer intero mattavelli buchi amplificati"/1(Out) -> Out1/1
  In1/1 -> " buffer intero mattavelli buchi amplificati"/1(e)

== system Filter_attivo/Controllo tensione/Controllo ripetitivo/Controllo ripetitivo con downsampling/Regolatore ripetitivo/ buffer intero fase zero ==
  e : Inport
  Add : Sum
  Delay1 : Delay  DelayLength=rit
  Delay2 : Delay  DelayLength=round((1/ro/f/Tc)-1-rit)
  Gain1 : Gain
  Gain2 : Gain  Gain=k_serie
  Q : DiscreteFir  Coefficients=[0.05 0.9 0.05]
  Scope : Subsystem  LoadFcn=plecs('sl', 300);  InitFcn=plecs('sl', 314);  StartFcn=plecs('sl', 308);  StopFcn=plecs('sl', 309);  mask{Settings=<binary blob, 424 chars, not shown>}
      mask init:
      | plecs('sl', 315);
      settings: CopyFcn=plecs('sl', 303);  DeleteFcn=plecs('sl', 305);  UndoDeleteFcn=plecs('sl', 306);  PreSaveFcn=plecs('sl', 311);  NameChangeFcn=plecs('sl', 310);  DestroyFcn=plecs('sl', 307);  OpenFcn=plecs('sl', 302);  ErrorFcn=plerrorfcn
      mask Display: plot([0.1 0.9 0.9 0.1 0.1], [0.9 0.9 0.5 0.5 0.9])
  Sum : Sum  Inputs=|++
  Out : Outport
  wires:
  Gain2/1 -> Add/2, Scope/2(2)
  Q/1 -> Delay1/1, Gain2/1
  Add/1 -> Scope/3(3), Out/1
  e/1 -> Add/1, Sum/1, Scope/1(1)
  Delay1/1 -> Gain1/1
  Delay2/1 -> Q/1
  Sum/1 -> Delay2/1
  Gain1/1 -> Sum/2

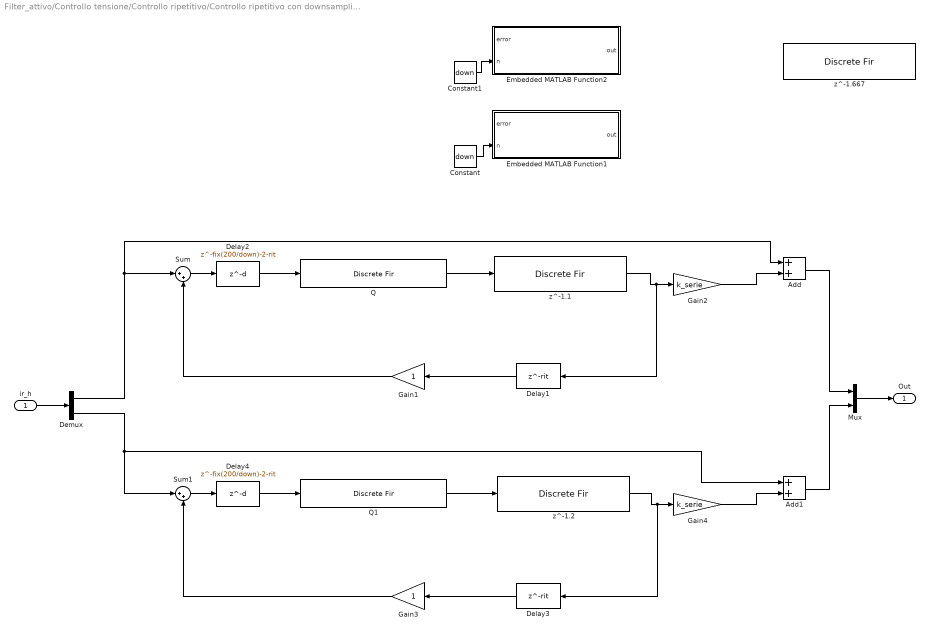
== system Filter_attivo/Controllo tensione/Controllo ripetitivo/Controllo ripetitivo con downsampling/Regolatore ripetitivo/ buffer intero fase zero-riduzione di 1 ==
  ir_h : Inport
  Add : Sum
  Add1 : Sum
  Constant : Constant  Value=down
  Constant1 : Constant  Value=down
  Delay1 : Delay  DelayLength=rit
  Delay2 : Delay  DelayLength=fix(200/down)-2-rit
  Delay3 : Delay  DelayLength=rit
  Delay4 : Delay  DelayLength=fix(200/down)-2-rit
  Demux : Demux  Outputs=2
  Embedded MATLAB Function1 : MATLAB Function  TreatAsAtomicUnit=on
  Embedded MATLAB Function2 : MATLAB Function  TreatAsAtomicUnit=on
  Gain1 : Gain
  Gain2 : Gain  Gain=k_serie
  Gain3 : Gain
  Gain4 : Gain  Gain=k_serie
  Mux : Mux  Inputs=2
  Q : DiscreteFir  Coefficients=[0.05 0.9 0.05]
  Q1 : DiscreteFir  Coefficients=[0.05 0.9 0.05]
  Sum : Sum  Inputs=|++
  Sum1 : Sum  Inputs=|++
  z^-1.1 : DiscreteFir  Coefficients="[ -0.0494  0.3704 0.7407 -0.0617]"
  z^-1.2 : DiscreteFir  Coefficients="[ -0.0494  0.3704 0.7407 -0.0617]"
  z^-1.667 : DiscreteFir  Coefficients="[ -0.0494  0.3704 0.7407 -0.0617]"
  Out : Outport
  wires:
  z^-1.2/1 -> Gain4/1, Delay3/1
  Q1/1 -> z^-1.2/1
  z^-1.1/1 -> Gain2/1, Delay1/1
  Q/1 -> z^-1.1/1
  Mux/1 -> Out/1
  Add1/1 -> Mux/2
  Add/1 -> Mux/1
  Demux/2 -> Sum1/1, Add1/1
  Constant1/1 -> Embedded MATLAB Function2/2(n)
  Gain3/1 -> Sum1/2
  Sum1/1 -> Delay4/1
  Delay4/1 -> Q1/1
  Delay3/1 -> Gain3/1
  Gain4/1 -> Add1/2
  Demux/1 -> Sum/1, Add/1
  ir_h/1 -> Demux/1
  Constant/1 -> Embedded MATLAB Function1/2(n)
  Gain1/1 -> Sum/2
  Sum/1 -> Delay2/1
  Delay2/1 -> Q/1
  Delay1/1 -> Gain1/1
  Gain2/1 -> Add/2

== system Filter_attivo/Controllo tensione/Controllo ripetitivo/Controllo ripetitivo con downsampling/Regolatore ripetitivo/ buffer intero fase zero-riduzione di 3 ==
  ir_h : Inport
  Add : Sum
  Add1 : Sum
  Delay1 : Delay  DelayLength=rit
  Delay2 : Delay  DelayLength=fix(200/down)-2-rit
  Delay3 : Delay  DelayLength=rit
  Delay4 : Delay  DelayLength=fix(200/down)-2-rit
  Demux : Demux  Outputs=2
  Gain1 : Gain
  Gain2 : Gain  Gain=k_serie
  Gain3 : Gain
  Gain4 : Gain  Gain=k_serie
  Mux : Mux  Inputs=2
  Q : DiscreteFir  Coefficients=[0.05 0.9 0.05]
  Q1 : DiscreteFir  Coefficients=[0.05 0.9 0.05]
  Sum : Sum  Inputs=|++
  Sum1 : Sum  Inputs=|++
  z^-1.1 : DiscreteFir  Coefficients="[ -0.0494  0.3704 0.7407 -0.0617]"
  z^-1.2 : DiscreteFir  Coefficients="[ -0.0494  0.3704 0.7407 -0.0617]"
  Out : Outport
  wires:
  Gain2/1 -> Add/2
  Delay1/1 -> Gain1/1
  Delay2/1 -> Q/1
  Sum/1 -> Delay2/1
  Gain1/1 -> Sum/2
  ir_h/1 -> Demux/1
  Demux/1 -> Add/1, Sum/1
  Gain4/1 -> Add1/2
  Delay3/1 -> Gain3/1
  Delay4/1 -> Q1/1
  Sum1/1 -> Delay4/1
  Gain3/1 -> Sum1/2
  Demux/2 -> Add1/1, Sum1/1
  Add/1 -> Mux/1
  Add1/1 -> Mux/2
  Mux/1 -> Out/1
  Q/1 -> z^-1.1/1
  z^-1.1/1 -> Delay1/1, Gain2/1
  Q1/1 -> z^-1.2/1
  z^-1.2/1 -> Delay3/1, Gain4/1

== system Filter_attivo/Controllo tensione/Controllo ripetitivo/Controllo ripetitivo con downsampling/Regolatore ripetitivo/ buffer intero mattavelli ==
  e : Inport
  Delay2 : Delay  DelayLength=round((1/ro/f/Tc)-1)
  Delay3 : Delay  DelayLength=round((1/ro/f/Tc)-rit)
  Gain2 : Gain  Gain=k_serie
  Q : DiscreteFir  Coefficients=[0.05 0.9 0.05]
  Sum : Sum  Inputs=|++
  Sum1 : Sum  Inputs=++|
  Sum2 : Sum
  Out : Outport
  wires:
  Sum/1 -> Sum1/1, Delay2/1
  Delay2/1 -> Q/1
  Q/1 -> Sum/2, Sum1/2
  e/1 -> Sum2/1, Sum/1
  Sum1/1 -> Delay3/1
  Delay3/1 -> Gain2/1
  Gain2/1 -> Sum2/2
  Sum2/1 -> Out/1

== system Filter_attivo/Controllo tensione/Controllo ripetitivo/Controllo ripetitivo con downsampling/Regolatore ripetitivo/ buffer intero mattavelli-riduzione di 3 ==
  e : Inport
  Delay1 : Delay  DelayLength=round((1/ro/f/Tc)-3-rit)
  Delay2 : Delay  DelayLength=round((1/ro/f/Tc)-2-rit)
  Gain2 : Gain  Gain=k_serie
  Q : DiscreteFir  Coefficients=[0.05 0.9 0.05]
  Sum : Sum  Inputs=|++
  Sum1 : Sum  Inputs=++|
  Sum2 : Sum
  z^-1.6 : DiscreteFir  Coefficients="[ -0.0494  0.3704 0.7407 -0.0617]"
  z^-1.667 : DiscreteFir  Coefficients="[ -0.0494  0.3704 0.7407 -0.0617]"
  Out : Outport
  wires:
  Sum2/1 -> Out/1
  Gain2/1 -> Sum2/2
  Delay2/1 -> z^-1.6/1
  Sum1/1 -> Delay2/1
  e/1 -> Sum/1, Sum2/1
  Q/1 -> z^-1.667/1
  Delay1/1 -> Q/1
  Sum/1 -> Delay1/1, Sum1/1
  z^-1.667/1 -> Sum1/2, Sum/2
  z^-1.6/1 -> Gain2/1

== system Filter_attivo/Controllo tensione/Controllo ripetitivo/Controllo ripetitivo con downsampling/Regolatore ripetitivo/ buffer metà fase zero ==
  e : Inport
  Add : Sum
  Delay1 : Delay  DelayLength=rit
  Delay2 : Delay  DelayLength=round((1/ro/f/Tc/down)-1-rit)
  Gain1 : Gain
  Gain2 : Gain  Gain=k_serie
  Q : DiscreteFir  Coefficients=[0.05 0.9 0.05]
  Scope : Subsystem  LoadFcn=plecs('sl', 300);  InitFcn=plecs('sl', 314);  StartFcn=plecs('sl', 308);  StopFcn=plecs('sl', 309);  mask{Settings=<binary blob, 424 chars, not shown>}
      mask init:
      | plecs('sl', 315);
      settings: CopyFcn=plecs('sl', 303);  DeleteFcn=plecs('sl', 305);  UndoDeleteFcn=plecs('sl', 306);  PreSaveFcn=plecs('sl', 311);  NameChangeFcn=plecs('sl', 310);  DestroyFcn=plecs('sl', 307);  OpenFcn=plecs('sl', 302);  ErrorFcn=plerrorfcn
      mask Display: plot([0.1 0.9 0.9 0.1 0.1], [0.9 0.9 0.5 0.5 0.9])
  Sum : Sum  Inputs=|--
  k_serie step : Subsystem  mask{k_serie_partenza=5, passo_t=0.6, passo_y=0}
      mask prompts: k_serie_partenza "partenza della costante"; passo_t "step dei tempi"; passo_y "step di costante"
  Out : Outport
  wires:
  Q/1 -> Delay1/1, Gain2/1
  Gain2/1 -> Add/2, Scope/2(2)
  Add/1 -> Scope/3(3), Out/1
  e/1 -> Add/1, Sum/1, Scope/1(1)
  Delay1/1 -> Gain1/1
  Delay2/1 -> Q/1
  Sum/1 -> Delay2/1
  Gain1/1 -> Sum/2

== system Filter_attivo/Controllo tensione/Controllo ripetitivo/Controllo ripetitivo con downsampling/Regolatore ripetitivo/ buffer metà fase zero-riduzione di 3 ==
  e : Inport
  Add : Sum
  Delay1 : Delay  DelayLength=rit
  Delay2 : Delay  DelayLength=round((1/ro/f/Tc/down)-2-rit)
  Gain1 : Gain
  Gain2 : Gain  Gain=k_serie
  Q : DiscreteFir  Coefficients=[0.05 0.9 0.05]
  Scope : Subsystem  LoadFcn=plecs('sl', 300);  InitFcn=plecs('sl', 314);  StartFcn=plecs('sl', 308);  StopFcn=plecs('sl', 309);  mask{Settings=<binary blob, 424 chars, not shown>}
      mask init:
      | plecs('sl', 315);
      settings: CopyFcn=plecs('sl', 303);  DeleteFcn=plecs('sl', 305);  UndoDeleteFcn=plecs('sl', 306);  PreSaveFcn=plecs('sl', 311);  NameChangeFcn=plecs('sl', 310);  DestroyFcn=plecs('sl', 307);  OpenFcn=plecs('sl', 302);  ErrorFcn=plerrorfcn
      mask Display: plot([0.1 0.9 0.9 0.1 0.1], [0.9 0.9 0.5 0.5 0.9])
  Sum : Sum  Inputs=|--
  k_serie step : Subsystem  mask{k_serie_partenza=5, passo_t=0.6, passo_y=0}
      mask prompts: k_serie_partenza "partenza della costante"; passo_t "step dei tempi"; passo_y "step di costante"
  z^-1.33 : DiscreteFir  Coefficients=[ -0.0617 0.7407 0.3704 -0.0494]
  Out : Outport
  wires:
  Gain1/1 -> Sum/2
  Sum/1 -> Delay2/1
  Delay2/1 -> Q/1
  Delay1/1 -> Gain1/1
  e/1 -> Scope/1(1), Sum/1, Add/1
  Add/1 -> Out/1, Scope/3(3)
  Gain2/1 -> Scope/2(2), Add/2
  Q/1 -> z^-1.33/1
  z^-1.33/1 -> Delay1/1, Gain2/1

== system Filter_attivo/Controllo tensione/Controllo ripetitivo/Controllo ripetitivo con downsampling/Regolatore ripetitivo/ buffer metà mattavelli ==
  e : Inport
  Add : Sum
  Delay2 : Delay  DelayLength=round((1/ro/f/Tc)-1)
  Delay3 : Delay  DelayLength=round((1/f/Tc/ro)-rit)
  Gain2 : Gain  Gain=k_serie
  Scope : Subsystem  LoadFcn=plecs('sl', 300);  InitFcn=plecs('sl', 314);  StartFcn=plecs('sl', 308);  StopFcn=plecs('sl', 309);  mask{Settings=<binary blob, 216 chars, not shown>}
      mask init:
      | plecs('sl', 315);
      settings: CopyFcn=plecs('sl', 303);  DeleteFcn=plecs('sl', 305);  UndoDeleteFcn=plecs('sl', 306);  PreSaveFcn=plecs('sl', 311);  NameChangeFcn=plecs('sl', 310);  DestroyFcn=plecs('sl', 307);  OpenFcn=plecs('sl', 302);  ErrorFcn=plerrorfcn
      mask Display: plot([0.1 0.9 0.9 0.1 0.1], [0.9 0.9 0.5 0.5 0.9])
  Sum : Sum  Inputs=|--
  Sum1 : Sum  Inputs=+-|
  Sum2 : Sum
  k_serie step : Subsystem  mask{k_serie_partenza=5, passo_t=0.6, passo_y=0}
      mask prompts: k_serie_partenza "partenza della costante"; passo_t "step dei tempi"; passo_y "step di costante"
  ritardo di 1.5 : DiscreteFir  Coefficients=[0.05 0.9 0.05]
  Out : Outport
  wires:
  Sum2/1 -> Out/1
  Gain2/1 -> Sum2/2
  Delay3/1 -> Gain2/1
  Sum1/1 -> Delay3/1
  e/1 -> Scope/1(1), Sum/1, Sum2/1
  ritardo di 1.5/1 -> Sum1/2, Sum/2
  Delay2/1 -> ritardo di 1.5/1
  Sum/1 -> Delay2/1, Sum1/1

== system Filter_attivo/Controllo tensione/Controllo ripetitivo/Controllo ripetitivo con downsampling/Regolatore ripetitivo/Scope ==
  1 : Inport
  " InputMux " : Subsystem
      mask Display: disp('Mux')
  " S-Function " : S-Function  FunctionName=plecs  SFunctionDeploymentMode=off  EnableBusSupport=off
  wires:
  1/1 -> " InputMux "/1(In1)
  " InputMux "/1(Out) -> " S-Function "/1

== system Filter_attivo/Controllo tensione/Controllo PR 10 kHz/Controllo risonante/FILTRO peaking inversa_prima/Scope/ InputMux  ==
  In1 : Inport
  Convert1 : DataTypeConversion  SaturateOnIntegerOverflow=on  RndMeth=Zero
  Mux : Mux  Inputs=1
  Out : Outport
  wires:
  Convert1/1 -> Mux/1
  In1/1 -> Convert1/1
  Mux/1 -> Out/1

== system Filter_attivo/Controllo tensione/Controllo PR 10 kHz/PLL_tempo_discreto/Subsystem/FILTRO peaking diretta_prima/Scope ==
  1 : Inport
  " InputMux " : Subsystem
      mask Display: disp('Mux')
  " S-Function " : S-Function  FunctionName=plecs  SFunctionDeploymentMode=off  EnableBusSupport=off
  wires:
  1/1 -> " InputMux "/1(In1)
  " InputMux "/1(Out) -> " S-Function "/1

== system Filter_attivo/Controllo tensione/Controllo PR 10 kHz/PLL_tempo_discreto/Subsystem/notch_prima_tensione/FILTRO peaking diretta_prima ==
  In2 : Inport
  Demux : Demux  Outputs=2
  Discrete Transfer Fcn : DiscreteTransferFcn  Numerator=cell2mat(Peaking_dir1_d(1,1).Num)  Denominator=cell2mat(Peaking_dir1_d(1,1).Den)
  Discrete Transfer Fcn1 : DiscreteTransferFcn  Numerator=cell2mat(Peaking_dir1_d(1,2).Num)  Denominator=cell2mat(Peaking_dir1_d(1,2).Den)
  Discrete Transfer Fcn2 : DiscreteTransferFcn  Numerator=cell2mat(Peaking_dir1_d(2,1).Num)  Denominator=cell2mat(Peaking_dir1_d(2,1).Den)
  Discrete Transfer Fcn3 : DiscreteTransferFcn  Numerator=cell2mat(Peaking_dir1_d(2,2).Num)  Denominator=cell2mat(Peaking_dir1_d(2,2).Den)
  Mux1 : Mux  Inputs=2
  Scope : Subsystem  LoadFcn=plecs('sl', 300);  InitFcn=plecs('sl', 314);  StartFcn=plecs('sl', 308);  StopFcn=plecs('sl', 309);  mask{Settings=<binary blob, 216 chars, not shown>}
      mask init:
      | plecs('sl', 315);
      settings: CopyFcn=plecs('sl', 303);  DeleteFcn=plecs('sl', 305);  UndoDeleteFcn=plecs('sl', 306);  PreSaveFcn=plecs('sl', 311);  NameChangeFcn=plecs('sl', 310);  DestroyFcn=plecs('sl', 307);  OpenFcn=plecs('sl', 302);  ErrorFcn=plerrorfcn
      mask Display: plot([0.1 0.9 0.9 0.1 0.1], [0.9 0.9 0.5 0.5 0.9])
  Sum3 : Sum  Inputs=|++
  Sum4 : Sum  Inputs=|++
  Out1 : Outport
  wires:
  Demux/1 -> Discrete Transfer Fcn2/1, Discrete Transfer Fcn/1
  Demux/2 -> Discrete Transfer Fcn1/1, Discrete Transfer Fcn3/1
  Discrete Transfer Fcn2/1 -> Sum4/1
  Sum4/1 -> Mux1/2
  Mux1/1 -> Out1/1
  Sum3/1 -> Mux1/1, Scope/1(1)
  Discrete Transfer Fcn/1 -> Sum3/1
  Discrete Transfer Fcn1/1 -> Sum3/2
  In2/1 -> Demux/1
  Discrete Transfer Fcn3/1 -> Sum4/2

== system Filter_attivo/Controllo tensione/Controllo ripetitivo/Controllo ripetitivo/Regolatore ripetitivo/ Ripetitivo sincrono/Scope ==
  1 : Inport
  2 : Inport  Port=2
  3 : Inport  Port=3
  " 1 " : DataTypeConversion  SaturateOnIntegerOverflow=on  RndMeth=Zero
  " 2 " : DataTypeConversion  SaturateOnIntegerOverflow=on  RndMeth=Zero
  " 3 " : DataTypeConversion  SaturateOnIntegerOverflow=on  RndMeth=Zero
  " InputMux " : Mux  Inputs=3
  " S-Function " : S-Function  FunctionName=plecs  SFunctionDeploymentMode=off  EnableBusSupport=off
  wires:
  " InputMux "/1 -> " S-Function "/1
  1/1 -> " 1 "/1
  " 1 "/1 -> " InputMux "/1
  2/1 -> " 2 "/1
  " 2 "/1 -> " InputMux "/2
  3/1 -> " 3 "/1
  " 3 "/1 -> " InputMux "/3

== system Filter_attivo/Controllo tensione/Controllo ripetitivo/Controllo ripetitivo/Regolatore ripetitivo/ buffer intero fase zero/Scope ==
  1 : Inport
  2 : Inport  Port=2
  3 : Inport  Port=3
  " 1 " : DataTypeConversion  SaturateOnIntegerOverflow=on  RndMeth=Zero
  " 2 " : DataTypeConversion  SaturateOnIntegerOverflow=on  RndMeth=Zero
  " 3 " : DataTypeConversion  SaturateOnIntegerOverflow=on  RndMeth=Zero
  " InputMux " : Mux  Inputs=3
  " S-Function " : S-Function  FunctionName=plecs  SFunctionDeploymentMode=off  EnableBusSupport=off
  wires:
  " 3 "/1 -> " InputMux "/3
  3/1 -> " 3 "/1
  " 2 "/1 -> " InputMux "/2
  2/1 -> " 2 "/1
  " 1 "/1 -> " InputMux "/1
  1/1 -> " 1 "/1
  " InputMux "/1 -> " S-Function "/1

== system Filter_attivo/Controllo tensione/Controllo ripetitivo/Controllo ripetitivo/Regolatore ripetitivo/ buffer intero fase zero/Subsystem ==
  errore : Inport
  Add : Sum
  Gain : Gain  Gain=g_disturbo
  Mux : Mux  Inputs=2
  Sine Wave : Sin  Frequency=f_disturbo*pi*2
  Sine Wave1 : Sin  Frequency=f_disturbo*pi*2  Phase=pi/2
  errore+disturbo : Outport
  wires:
  Sine Wave/1 -> Mux/2
  Add/1 -> errore+disturbo/1
  Sine Wave1/1 -> Mux/1
  errore/1 -> Add/1
  Mux/1 -> Gain/1
  Gain/1 -> Add/2

== system Filter_attivo/Controllo tensione/Controllo ripetitivo/Controllo ripetitivo/Regolatore ripetitivo/ buffer intero fase zero1/Scope ==
  1 : Inport
  2 : Inport  Port=2
  3 : Inport  Port=3
  " 1 " : DataTypeConversion  SaturateOnIntegerOverflow=on  RndMeth=Zero
  " 2 " : DataTypeConversion  SaturateOnIntegerOverflow=on  RndMeth=Zero
  " 3 " : DataTypeConversion  SaturateOnIntegerOverflow=on  RndMeth=Zero
  " InputMux " : Mux  Inputs=3
  " S-Function " : S-Function  FunctionName=plecs  SFunctionDeploymentMode=off  EnableBusSupport=off
  wires:
  " InputMux "/1 -> " S-Function "/1
  1/1 -> " 1 "/1
  " 1 "/1 -> " InputMux "/1
  2/1 -> " 2 "/1
  " 2 "/1 -> " InputMux "/2
  3/1 -> " 3 "/1
  " 3 "/1 -> " InputMux "/3

== system Filter_attivo/Controllo tensione/Controllo ripetitivo/Controllo ripetitivo/Regolatore ripetitivo/ buffer intero feedforward/Scope ==
  1 : Inport
  " InputMux " : Subsystem
      mask Display: disp('Mux')
  " S-Function " : S-Function  FunctionName=plecs  SFunctionDeploymentMode=off  EnableBusSupport=off
  wires:
  1/1 -> " InputMux "/1(In1)
  " InputMux "/1(Out) -> " S-Function "/1

== system Filter_attivo/Controllo tensione/Controllo ripetitivo/Controllo ripetitivo/Regolatore ripetitivo/ buffer intero feedforward/Scope1 ==
  1 : Inport
  " InputMux " : Subsystem
      mask Display: disp('Mux')
  " S-Function " : S-Function  FunctionName=plecs  SFunctionDeploymentMode=off  EnableBusSupport=off
  wires:
  " InputMux "/1(Out) -> " S-Function "/1
  1/1 -> " InputMux "/1(In1)

== system Filter_attivo/Controllo tensione/Controllo ripetitivo/Controllo ripetitivo/Regolatore ripetitivo/ buffer intero feedforward/Subsystem ==
  errore : Inport
  Add : Sum
  Gain : Gain  Gain=g_disturbo
  Mux : Mux  Inputs=2
  Sine Wave : Sin  Frequency=f_disturbo*pi*2
  Sine Wave1 : Sin  Frequency=f_disturbo*pi*2  Phase=pi/2
  errore+disturbo : Outport
  wires:
  Sine Wave/1 -> Mux/2
  Add/1 -> errore+disturbo/1
  Sine Wave1/1 -> Mux/1
  errore/1 -> Add/1
  Mux/1 -> Gain/1
  Gain/1 -> Add/2

== system Filter_attivo/Controllo tensione/Controllo ripetitivo/Controllo ripetitivo/Regolatore ripetitivo/ buffer metà fase zero/Scope ==
  1 : Inport
  2 : Inport  Port=2
  3 : Inport  Port=3
  " 1 " : DataTypeConversion  SaturateOnIntegerOverflow=on  RndMeth=Zero
  " 2 " : DataTypeConversion  SaturateOnIntegerOverflow=on  RndMeth=Zero
  " 3 " : DataTypeConversion  SaturateOnIntegerOverflow=on  RndMeth=Zero
  " InputMux " : Mux  Inputs=3
  " S-Function " : S-Function  FunctionName=plecs  SFunctionDeploymentMode=off  EnableBusSupport=off
  wires:
  " 3 "/1 -> " InputMux "/3
  3/1 -> " 3 "/1
  " 2 "/1 -> " InputMux "/2
  2/1 -> " 2 "/1
  " 1 "/1 -> " InputMux "/1
  1/1 -> " 1 "/1
  " InputMux "/1 -> " S-Function "/1

== system Filter_attivo/Controllo tensione/Controllo ripetitivo/Controllo ripetitivo/Regolatore ripetitivo/ buffer metà feedforward/Scope ==
  1 : Inport
  " InputMux " : Subsystem
      mask Display: disp('Mux')
  " S-Function " : S-Function  FunctionName=plecs  SFunctionDeploymentMode=off  EnableBusSupport=off
  wires:
  " InputMux "/1(Out) -> " S-Function "/1
  1/1 -> " InputMux "/1(In1)

== system Filter_attivo/Controllo tensione/Controllo ripetitivo/Controllo ripetitivo/Regolatore ripetitivo/ buffer metà feedforward/Subsystem ==
  errore : Inport
  Add : Sum
  Gain : Gain  Gain=g_disturbo
  Mux : Mux  Inputs=2
  Sine Wave : Sin  Frequency=f_disturbo*pi*2
  Sine Wave1 : Sin  Frequency=f_disturbo*pi*2  Phase=pi/2
  errore+disturbo : Outport
  wires:
  Sine Wave/1 -> Mux/2
  Add/1 -> errore+disturbo/1
  Sine Wave1/1 -> Mux/1
  errore/1 -> Add/1
  Mux/1 -> Gain/1
  Gain/1 -> Add/2

== system Filter_attivo/Controllo tensione/Controllo ripetitivo/Controllo ripetitivo/Regolatore ripetitivo/Ripetitivo Modulazione AM/Banco di ripetitivi ==
  In1 : Inport
  Enable : EnablePort  StatesWhenEnabling=reset
  Subsystem : Subsystem  mask{abilitatore5=1, abilitatore7=1, abilitatore11=1, abilitatore13=0, abilitatore17=0, abilitatore19=0}
      mask prompts: abilitatore5 "5^a armonica"; abilitatore7 "7^a armonica"; abilitatore11 "11^ armonica"; abilitatore13 "13^ armonica"; abilitatore17 "17^ armonica"; abilitatore19 "19^ armonica"
  rep_comp 1 : Subsystem  mask{ro=5+(f_am/50), g_interno=8, rit=2}
      mask prompts: ro "Harmonic order"; g_interno "guadagno serie"; rit "ritardo inverter"
  rep_comp 2 : Subsystem  mask{ro=7+(f_am/50), g_interno=1.9, rit=2}
      mask prompts: ro "Harmonic order"; g_interno "guadagno serie"; rit "ritardo inverter"
  rep_comp 3 : Subsystem  mask{ro=11+(f_am/50), g_interno=1, rit=2}
      mask prompts: ro "Harmonic order"; g_interno "guadagno serie"; rit "ritardo inverter"
  rep_comp 4 : Subsystem  mask{ro=13+(f_am/50), g_interno=1, rit=2}
      mask prompts: ro "Harmonic order"; g_interno "guadagno serie"; rit "ritardo inverter"
  rep_comp 5 : Subsystem  mask{ro=17+(f_am/50), g_interno=0.5, rit=2}
      mask prompts: ro "Harmonic order"; g_interno "guadagno serie"; rit "ritardo inverter"
  rep_comp 6 : Subsystem  mask{ro=19+(f_am/50), g_interno=0.5, rit=2}
      mask prompts: ro "Harmonic order"; g_interno "guadagno serie"; rit "ritardo inverter"
  Out1 : Outport
  wires:
  In1/1 -> rep_comp 3/1(In1), rep_comp 4/1(In1), rep_comp 6/1(In1), rep_comp 5/1(In1), rep_comp 2/1(In1), rep_comp 1/1(In1)
  Subsystem/1(Out1) -> Out1/1
  rep_comp 1/1(Out1) -> Subsystem/1(In1)
  rep_comp 2/1(Out1) -> Subsystem/2(In2)
  rep_comp 3/1(Out1) -> Subsystem/3(In3)
  rep_comp 4/1(Out1) -> Subsystem/4(In4)
  rep_comp 5/1(Out1) -> Subsystem/5(In5)
  rep_comp 6/1(Out1) -> Subsystem/6(In6)

== system Filter_attivo/Controllo tensione/Controllo ripetitivo/Controllo ripetitivo/Regolatore ripetitivo/Ripetitivo Modulazione AM/Banco notch 5_7_AM ==
  In2 : Inport
  Enable : EnablePort  StatesWhenEnabling=reset
  Demux1 : Demux  Outputs=2
  Mux1 : Mux  Inputs=2
  notch_demodulazione_5_1 : Subsystem
  notch_demodulazione_5_7 : Subsystem
  Out1 : Outport
  wires:
  Mux1/1 -> Out1/1
  Demux1/1 -> notch_demodulazione_5_7/1(In1)
  notch_demodulazione_5_7/1(Out1) -> Mux1/1
  notch_demodulazione_5_1/1(Out1) -> Mux1/2
  In2/1 -> Demux1/1
  Demux1/2 -> notch_demodulazione_5_1/1(In1)

== system Filter_attivo/Controllo tensione/Controllo ripetitivo/Controllo ripetitivo/Regolatore ripetitivo/Ripetitivo Modulazione AM/Integratore discreto con reset a 2*pi ==
  omega : Inport
  Add : Sum
  Compare To Zero : simulink/Logic and Bit Operations/Compare To Zero  relop=>  OutDataTypeStr=uint8  ZeroCross=off
  Constant : Constant  Value=2*pi
  Constant1 : Constant  Value=-2*pi
  Constant2 : Constant  Value=-2*pi
  Constant3 : Constant  Value=2*pi
  Discrete-Time Integrator : DiscreteIntegrator  ExternalReset=rising  InitialConditionSource=external  SampleTime=-1  ShowStatePort=on  ICPrevOutput=DiscIntNeverNeededParam  ICPrevScaledInput=DiscIntNeverNeededParam
  Logical Operator2 : Logic  Operator=OR  AllPortsSameDT=off  OutDataTypeStr=boolean
  Relational Operator : RelationalOperator  Operator=<=  OutDataTypeStr=boolean  RndMeth=Nearest
  Relational Operator1 : RelationalOperator  Operator=<=  OutDataTypeStr=boolean  RndMeth=Nearest
  Switch : Switch  Threshold=0.5
  teta : Outport
  wires:
  Logical Operator2/1 -> Discrete-Time Integrator/2
  Relational Operator/1 -> Logical Operator2/1
  Relational Operator1/1 -> Logical Operator2/2
  Discrete-Time Integrator/State -> Add/1, Compare To Zero/1, Relational Operator1/1, Relational Operator/2
  Constant/1 -> Relational Operator/1
  Constant1/1 -> Relational Operator1/2
  omega/1 -> Discrete-Time Integrator/1
  Discrete-Time Integrator/1 -> teta/1
  Constant2/1 -> Switch/1
  Constant3/1 -> Switch/3
  Switch/1 -> Add/2
  Compare To Zero/1 -> Switch/2
  Add/1 -> Discrete-Time Integrator/3

== system Filter_attivo/Controllo tensione/Controllo ripetitivo/Controllo ripetitivo/Regolatore ripetitivo/Ripetitivo Modulazione AM/Scope ==
  1 : Inport
  2 : Inport  Port=2
  3 : Inport  Port=3
  " 1 " : DataTypeConversion  SaturateOnIntegerOverflow=on  RndMeth=Zero
  " 2 " : DataTypeConversion  SaturateOnIntegerOverflow=on  RndMeth=Zero
  " 3 " : DataTypeConversion  SaturateOnIntegerOverflow=on  RndMeth=Zero
  " InputMux " : Mux  Inputs=3
  " S-Function " : S-Function  FunctionName=plecs  SFunctionDeploymentMode=off  EnableBusSupport=off
  wires:
  " InputMux "/1 -> " S-Function "/1
  1/1 -> " 1 "/1
  " 1 "/1 -> " InputMux "/1
  2/1 -> " 2 "/1
  " 2 "/1 -> " InputMux "/2
  3/1 -> " 3 "/1
  " 3 "/1 -> " InputMux "/3

== system Filter_attivo/Controllo tensione/Controllo ripetitivo/Controllo ripetitivo/Regolatore ripetitivo/Ripetitivo Modulazione AM/Scope1 ==
  1 : Inport
  2 : Inport  Port=2
  " 1 " : DataTypeConversion  SaturateOnIntegerOverflow=on  RndMeth=Zero
  " 2 " : DataTypeConversion  SaturateOnIntegerOverflow=on  RndMeth=Zero
  " InputMux " : Mux  Inputs=2
  " S-Function " : S-Function  FunctionName=plecs  SFunctionDeploymentMode=off  EnableBusSupport=off
  wires:
  " InputMux "/1 -> " S-Function "/1
  1/1 -> " 1 "/1
  " 1 "/1 -> " InputMux "/1
  2/1 -> " 2 "/1
  " 2 "/1 -> " InputMux "/2
